simulink model "hydraulicCylinder_1"  (R2025b)
settings: Solver=VariableStepAuto  StartTime=0.0  StopTime=30  RelTol=1e-3
InitFcn:
  | hyd_parameter
undefined symbols (not defined in the file or in its folder): cyl, valve
libraries: SignalEditorBlockLib x3, slpidlib x1, simulink x1
settings Model: LastModifiedBy=binh.le

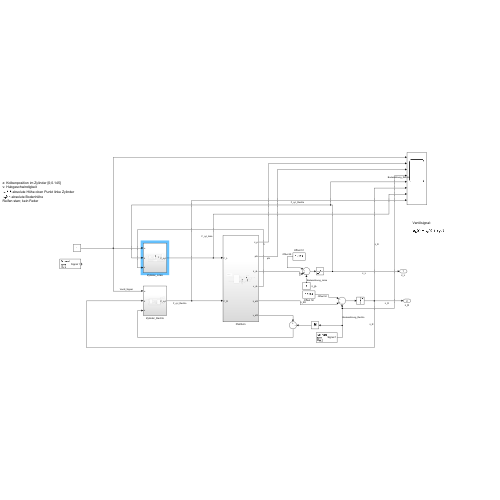
[thumbnail: Simulink's stored preview of the top-level diagram]
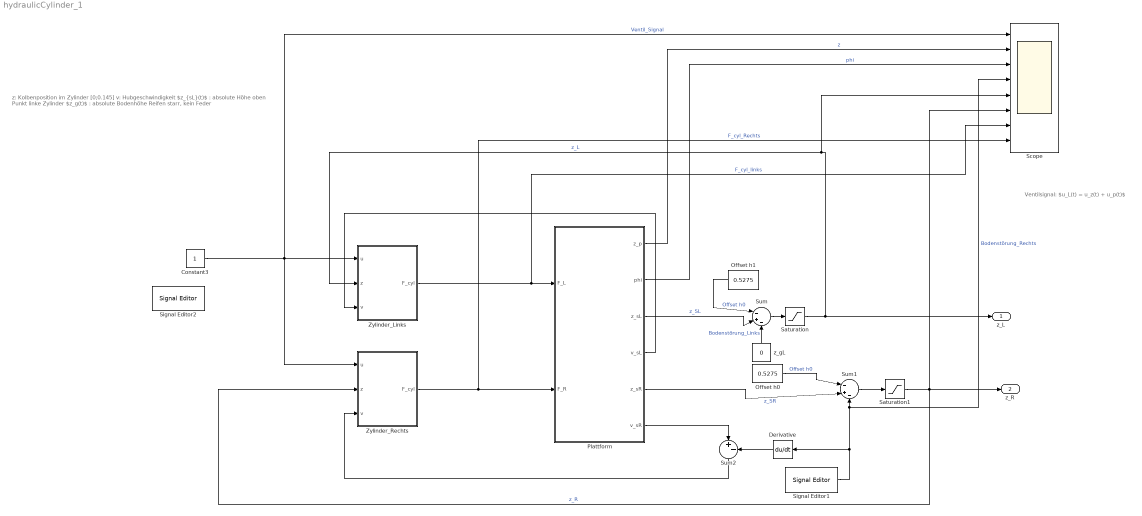
== system hydraulicCylinder_1 ==
  note: z: Kolbenposition im Zylinder [0;0.145]
      | v: Hubgeschwindigkeit
      | $z_{sL}(t)$ : absolute Höhe oben Punkt linke Zylinder
      | $z_g(t)$ : absolute Bodenhöhe
      | Reifen starr, kein Feder
  note: Ventilsignal:
      |
      | $u_L(t) = u_z(t) + u_p(t)$
  Constant3 : Constant
  Derivative : Derivative
  Offset h0 : Constant  Value=0.5275
  Offset h1 : Constant  Value=0.5275
  Plattform : Subsystem
  Saturation : Saturate  UpperLimit=0.145  LowerLimit=0
  Saturation1 : Saturate  UpperLimit=0.145  LowerLimit=0
  Scope : Scope  NumInputPorts=8
      settings: ActiveDisplayString=7  ActiveDisplayYMinimum=-28869.174120408497  ActiveDisplayYMaximum=66545.684568252938
  Signal Editor1 : SignalEditorBlockLib/Signal Editor  FileName=W:\BINH_MATLAB\bodenstörung.mat  ActiveScenario=Scenario  ActiveSignal=Signal 1  IsBus=off  OutputBusObjectStr=Bus: BusObject  SampleTime=0  ZeroCross=off  OutputAfterFinalValue=Setting to zero  Unit=inherit  PreserveSignalName=on  ApplySigPropsToAllScenarios=on  ApplySigPropsToAllSignals=off  SignalPropertySource=Dialog parameters
  Signal Editor2 : SignalEditorBlockLib/Signal Editor  FileName=signal.mat  ActiveScenario=Scenario  ActiveSignal=Signal 1  IsBus=off  OutputBusObjectStr=Bus: BusObject  SampleTime=0  ZeroCross=off  OutputAfterFinalValue=Setting to zero  Unit=inherit  PreserveSignalName=on  ApplySigPropsToAllScenarios=on  ApplySigPropsToAllSignals=off  SignalPropertySource=Dialog parameters
  Sum : Sum  Inputs=|-+-
  Sum1 : Sum  Inputs=|-+-
  Sum2 : Sum  Inputs=|+-
  Zylinder_Links : Subsystem
  Zylinder_Rechts : Subsystem
  z_gL : Constant  Value=0
  z_L : Outport
  z_R : Outport  Port=2
  wires:
  Zylinder_Links/1(F_cyl) -> Scope/7, Plattform/1(F_L)  "F_cyl_links"
  Zylinder_Rechts/1(F_cyl) -> Scope/8, Plattform/2(F_R)  "F_cyl_Rechts"
  Plattform/3(z_sL) -> Sum/2  "z_SL"
  z_gL/1 -> Sum/3  "Bodenstörung_Links"
  Sum/1 -> Saturation/1
  Constant3/1 -> Zylinder_Rechts/1(u), Scope/1, Zylinder_Links/1(u)  "Ventil_Signal"
  Plattform/1(z_p) -> Scope/2  "z"
  Plattform/2(phi) -> Scope/3  "phi"
  Plattform/5(z_sR) -> Sum1/2  "z_SR"
  Sum1/1 -> Saturation1/1
  Plattform/4(v_sL) -> Zylinder_Links/3(v)
  Saturation/1 -> Scope/5, Zylinder_Links/2(z), z_L/1  "z_L"
  Saturation1/1 -> Scope/6, Zylinder_Rechts/2(z), z_R/1  "z_R"
  Signal Editor1/1 -> Derivative/1, Scope/4, Sum1/3  "Bodenstörung_Rechts"
  Derivative/1 -> Sum2/2
  Plattform/6(v_sR) -> Sum2/1
  Sum2/1 -> Zylinder_Rechts/3(v)
  Offset h0/1 -> Sum1/1  "Offset h0"
  Offset h1/1 -> Sum/1  "Offset h0"

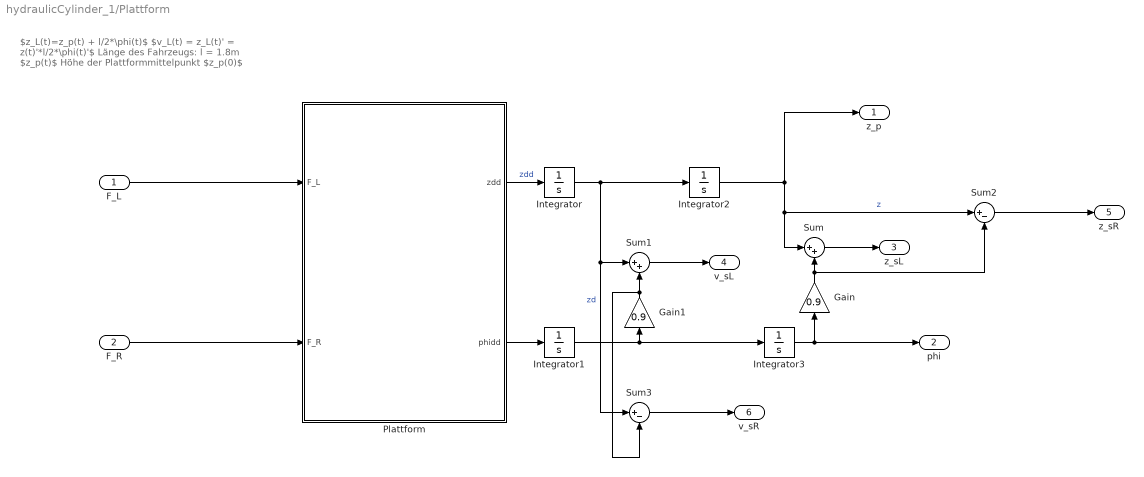
== system hydraulicCylinder_1/Plattform ==
  note: $z_L(t)=z_p(t) + l/2*\phi(t)$
      | $v_L(t) = z_L(t)' = z(t)'*l/2*\phi(t)'$
      | Länge des Fahrzeugs: l = 1.8m
      | $z_p(t)$ Höhe der Plattformmittelpunkt
      | $z_p(0)$
  F_L : Inport
  F_R : Inport  Port=2
  Gain : Gain  Gain=0.9
  Gain1 : Gain  Gain=0.9
  Integrator : Integrator
  Integrator1 : Integrator
  Integrator2 : Integrator  InitialCondition=0.6
  Integrator3 : Integrator
  Plattform : MATLAB Function  TreatAsAtomicUnit=on
  Sum : Sum  Inputs=|++
  Sum1 : Sum  Inputs=|++
  Sum2 : Sum  Inputs=|+-
  Sum3 : Sum  Inputs=|+-
  z_p : Outport
  phi : Outport  Port=2
  z_sL : Outport  Port=3
  v_sL : Outport  Port=4
  z_sR : Outport  Port=5
  v_sR : Outport  Port=6
  wires:
  Integrator/1 -> Sum3/1, Sum1/1, Integrator2/1  "zd"
  Integrator2/1 -> Sum/1, Sum2/1, z_p/1  "z"
  Plattform/2(phidd) -> Integrator1/1
  Plattform/1(zdd) -> Integrator/1  "zdd"
  F_L/1 -> Plattform/1(F_L)
  Integrator1/1 -> Gain1/1, Integrator3/1
  F_R/1 -> Plattform/2(F_R)
  Integrator3/1 -> phi/1, Gain/1
  Gain/1 -> Sum2/2, Sum/2
  Sum/1 -> z_sL/1
  Gain1/1 -> Sum3/2, Sum1/2
  Sum1/1 -> v_sL/1
  Sum2/1 -> z_sR/1
  Sum3/1 -> v_sR/1

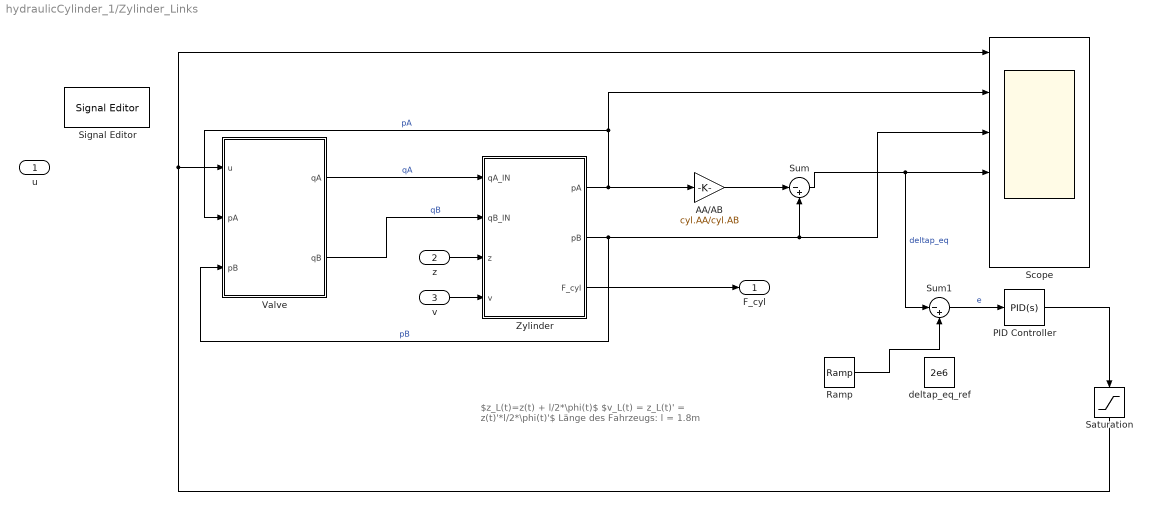
== system hydraulicCylinder_1/Zylinder_Links ==
  note: $z_L(t)=z(t) + l/2*\phi(t)$
      | $v_L(t) = z_L(t)' = z(t)'*l/2*\phi(t)'$
      | Länge des Fahrzeugs: l = 1.8m
  u : Inport
  z : Inport  Port=2
  v : Inport  Port=3
  AA/AB : Gain  Gain=cyl.AA/cyl.AB
  PID Controller : slpidlib/PID Controller  Controller=PID  Form=Parallel  TimeDomain=Continuous-time  UseExternalTs=off  SampleTime=-1  IntegratorMethod=Forward Euler  FilterMethod=Forward Euler  ControllerParametersSource=internal  P=4e-7  I=1e-7  UseKiTs=off  D=0  UseExternalDerivativeSource=off  N=100  UseFilter=on  TunerSelectOption=Transfer Function Based (PID Tuner App)  InitialConditionSource=internal  InitialConditionForIntegrator=0  InitialConditionForFilter=0  DifferentiatorICPrevScaledInput=0  ExternalReset=none  TrackingMode=off  Kt=1  LimitOutput=on  SatLimitsSource=internal  UpperSaturationLimit=1  LowerSaturationLimit=-1  LinearizeAsGain=on  AntiWindupMode=back-calculation  Kb=50  LimitIntegrator=off  UpperIntegratorSaturationLimit=inf  LowerIntegratorSaturationLimit=-inf  POutMin=[]  POutMax=[]  IOutMin=[]  IOutMax=[]  DOutMin=[]  DOutMax=[]  NOutMin=[]  NOutMax=[]  SumOutMin=[]  SumOutMax=[]  SaturationOutMin=[]  SaturationOutMax=[]  PParamMin=[]  PParamMax=[]  IParamMin=[]  IParamMax=[]  DParamMin=[]  DParamMax=[]  NParamMin=[]  NParamMax=[]  KbParamMin=[]  KbParamMax=[]  KtParamMin=[]  KtParamMax=[]  KbOutMin=[]  KbOutMax=[]  KtOutMin=[]  KtOutMax=[]  IntegratorOutMin=[]  IntegratorOutMax=[]  FilterOutMin=[]  FilterOutMax=[]  SumI1OutMin=[]  SumI1OutMax=[]  SumI2OutMin=[]  SumI2OutMax=[]  SumI3OutMin=[]  SumI3OutMax=[]  SumI4OutMin=[]  SumI4OutMax=[]  SumDOutMin=[]  SumDOutMax=[]  DifferentiatorOutMin=[]  DifferentiatorOutMax=[]  FilterDiffOutCoefMin=[]  FilterDiffOutCoefMax=[]  ReciprocalOutMin=[]  ReciprocalOutMax=[]  SumDenOutMin=[]  SumDenOutMax=[]  SumNumOutMin=[]  SumNumOutMax=[]  DivideOutMin=[]  DivideOutMax=[]  UdiffTsProdOutMin=[]  UdiffTsProdOutMax=[]  NTsProdOutMin=[]  NTsProdOutMax=[]  UintegralTsProdOutMin=[]  UintegralTsProdOutMax=[]  UngainTsProdOutMin=[]  UngainTsProdOutMax=[]  ClampingZeroOutDataTypeStr=Inherit: Inherit via back propagation  ClampingZeroOutMin=[]  ClampingZeroOutMax=[]  FilterDenConstantOutDataTypeStr=Inherit: Inherit via back propagation  FilterDenConstantOutMin=[]  FilterDenConstantOutMax=[]  PCopyOutDataTypeStr=Inherit: Inherit via back propagation  PCopyOutMin=[]  PCopyOutMax=[]  NCopyOutDataTypeStr=Inherit: Inherit via back propagation  NCopyOutMin=[]  NCopyOutMax=[]  IntegratorContinuousStateAttributes=''  IntegratorStateMustResolveToSignalObject=off  IntegratorRTWStateStorageClass=Auto  FilterContinuousStateAttributes=''  FilterStateMustResolveToSignalObject=off  FilterRTWStateStorageClass=Auto  ParallelPVariant=InternalParameters  IdealPVariant=Disabled  IVariant=InternalParameters  DVariant=InternalParameters  IntegratorVariant=Continuous  SatVariant=Enabled  AWVariant=BackCalculation  PCopyVariant=Disabled  TRVariant=Disabled  FdbkBlocksVariant=Forward  IdealPFdbkVariant=Disabled  SatFdbkVariant=Disabled  DerivativeFilterVariant=ContFilter  NVariant=InternalParameters  NCopyVariant=Disabled  FilterICVariant=InternalICsFilter  IntegratorICVariant=InternalICs  ExternalResetVariant=Disabled  TRSumVariant=Passthrough  SumFdbkVariant=Disabled  SumVariant=Sum_PID  TsampFilterVariant=InternalTs  TsampNgainVariant=Passthrough  TsampIntegralVariant=Disabled_SignalSpec  ExternalSaturationOutDataTypeStr=Inherit: Same as second input  DerivativeSourceVariant=ErrorSignal  PreIntVariant=InternalPreInt
  Ramp : simulink/Sources/Ramp  slope=2e6  start=2  InitialOutput=0
  Saturation : Saturate  UpperLimit=1  LowerLimit=-1
  Scope : Scope  NumInputPorts=6
      settings: ActiveDisplayYMinimum=-1.25  ActiveDisplayYMaximum=1.25
  Signal Editor : SignalEditorBlockLib/Signal Editor  FileName=signal.mat  ActiveScenario=Scenario  ActiveSignal=Signal 1  IsBus=off  OutputBusObjectStr=Bus: BusObject  SampleTime=0  ZeroCross=off  OutputAfterFinalValue=Setting to zero  Unit=inherit  PreserveSignalName=on  ApplySigPropsToAllScenarios=on  ApplySigPropsToAllSignals=off  SignalPropertySource=Dialog parameters
  Sum : Sum  Inputs=|-+
  Sum1 : Sum  Inputs=|-+
  Valve : Subsystem
  Zylinder : Subsystem
  deltap_eq_ref : Constant  Value=2e6
  F_cyl : Outport
  wires:
  PID Controller/1 -> Saturation/1
  z/1 -> Zylinder/3(z)
  Zylinder/2(pB) -> Sum/2, Scope/3, Valve/3(pB)  "pB"
  v/1 -> Zylinder/4(v)
  Zylinder/3(F_cyl) -> F_cyl/1
  Zylinder/1(pA) -> Valve/2(pA), Scope/2, AA/AB/1  "pA"
  Valve/1(qA) -> Zylinder/1(qA_IN)  "qA"
  Valve/2(qB) -> Zylinder/2(qB_IN)  "qB"
  Sum/1 -> Scope/4, Sum1/1  "deltap_eq"
  AA/AB/1 -> Sum/1
  Ramp/1 -> Sum1/2
  Sum1/1 -> PID Controller/1  "e"
  Saturation/1 -> Scope/1, Valve/1(u)

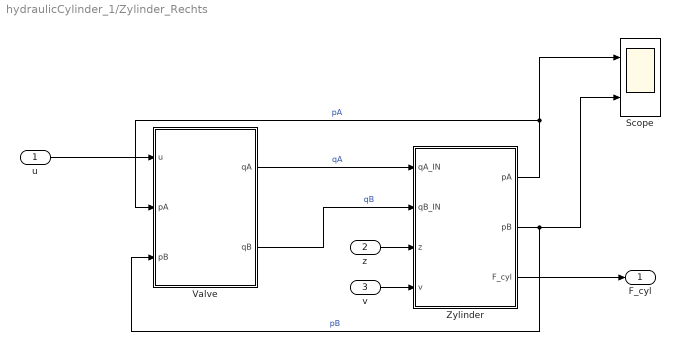
== system hydraulicCylinder_1/Zylinder_Rechts ==
  u : Inport
  z : Inport  Port=2
  v : Inport  Port=3
  Scope : Scope  NumInputPorts=2
      settings: ActiveDisplayYMinimum=-1  ActiveDisplayYMaximum=1  DataLoggingVariableName=ScopeData2
  Valve : Subsystem
  Zylinder : Subsystem
  F_cyl : Outport
  wires:
  u/1 -> Valve/1(u)
  z/1 -> Zylinder/3(z)
  Zylinder/2(pB) -> Scope/2, Valve/3(pB)  "pB"
  v/1 -> Zylinder/4(v)
  Zylinder/3(F_cyl) -> F_cyl/1
  Zylinder/1(pA) -> Scope/1, Valve/2(pA)  "pA"
  Valve/1(qA) -> Zylinder/1(qA_IN)  "qA"
  Valve/2(qB) -> Zylinder/2(qB_IN)  "qB"

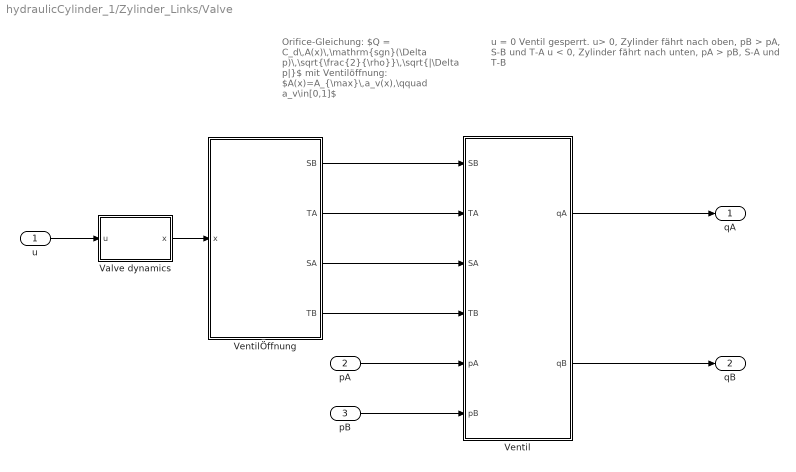
== system hydraulicCylinder_1/Zylinder_Links/Valve ==
  note: Orifice-Gleichung:
      | $Q = C_d\,A(x)\,\mathrm{sgn}(\Delta p)\,\sqrt{\frac{2}{\rho}}\,\sqrt{|\Delta p|}$
      | mit Ventilöffnung:
      | $A(x)=A_{\max}\,a_v(x),\qquad a_v\in[0,1]$
  note: u = 0 Ventil gesperrt.
      | u> 0, Zylinder fährt nach oben, pB > pA, S-B und T-A
      | u < 0, Zylinder fährt nach unten, pA > pB, S-A und T-B
  u : Inport
  pA : Inport  Port=2
  pB : Inport  Port=3
  Valve dynamics : Subsystem
  Ventil : MATLAB Function  TreatAsAtomicUnit=on
  VentilÖffnung : MATLAB Function  TreatAsAtomicUnit=on
  qA : Outport
  qB : Outport  Port=2
  wires:
  Ventil/1(qA) -> qA/1
  Ventil/2(qB) -> qB/1
  pB/1 -> Ventil/6(pB)
  pA/1 -> Ventil/5(pA)
  u/1 -> Valve dynamics/1(u)
  Valve dynamics/1(x) -> VentilÖffnung/1(x)
  VentilÖffnung/3(SA) -> Ventil/3(SA)
  VentilÖffnung/2(TA) -> Ventil/2(TA)
  VentilÖffnung/1(SB) -> Ventil/1(SB)
  VentilÖffnung/4(TB) -> Ventil/4(TB)

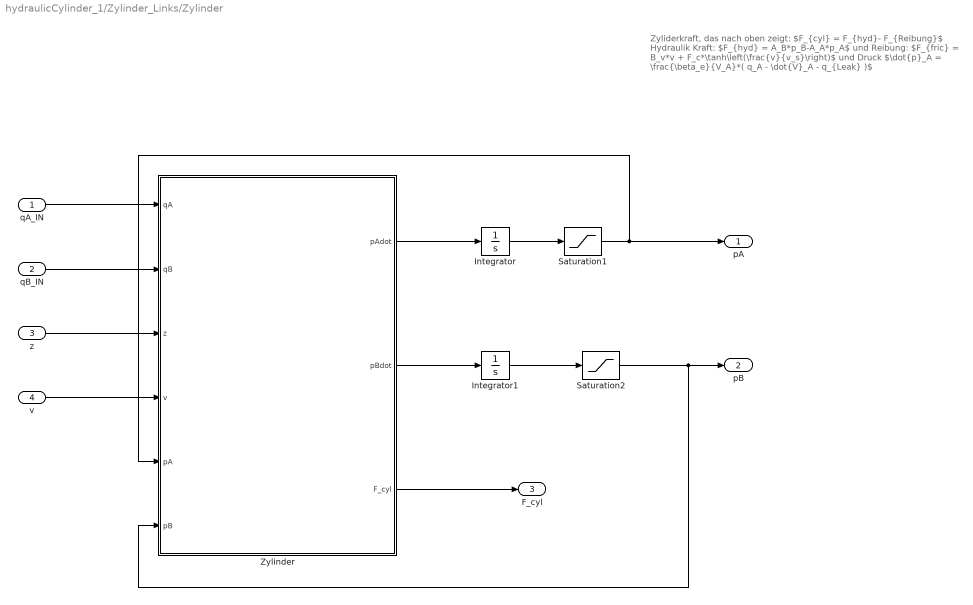
== system hydraulicCylinder_1/Zylinder_Links/Zylinder ==
  note: Zyliderkraft, das nach oben zeigt:
      | $F_{cyl} = F_{hyd}- F_{Reibung}$
      | Hydraulik Kraft:
      | $F_{hyd} = A_B*p_B-A_A*p_A$
      | und Reibung:
      | $F_{fric} = B_v*v + F_c*\tanh\left(\frac{v}{v_s}\right)$
      | und Druck
      | $\dot{p}_A = \frac{\beta_e}{V_A}*( q_A - \dot{V}_A - q_{Leak} )$
  qA_IN : Inport
  qB_IN : Inport  Port=2
  z : Inport  Port=3
  v : Inport  Port=4
  Integrator : Integrator  InitialCondition=valve.pT
  Integrator1 : Integrator  InitialCondition=9e6
  Saturation1 : Saturate  UpperLimit=cyl.pMax  LowerLimit=cyl.pMin
  Saturation2 : Saturate  UpperLimit=cyl.pMax  LowerLimit=cyl.pMin
  Zylinder : MATLAB Function  TreatAsAtomicUnit=on
  pA : Outport
  pB : Outport  Port=2
  F_cyl : Outport  Port=3
  wires:
  v/1 -> Zylinder/4(v)
  z/1 -> Zylinder/3(z)
  qA_IN/1 -> Zylinder/1(qA)
  qB_IN/1 -> Zylinder/2(qB)
  Zylinder/1(pAdot) -> Integrator/1
  Zylinder/2(pBdot) -> Integrator1/1
  Zylinder/3(F_cyl) -> F_cyl/1
  Integrator/1 -> Saturation1/1
  Integrator1/1 -> Saturation2/1
  Saturation1/1 -> Zylinder/5(pA), pA/1
  Saturation2/1 -> Zylinder/6(pB), pB/1

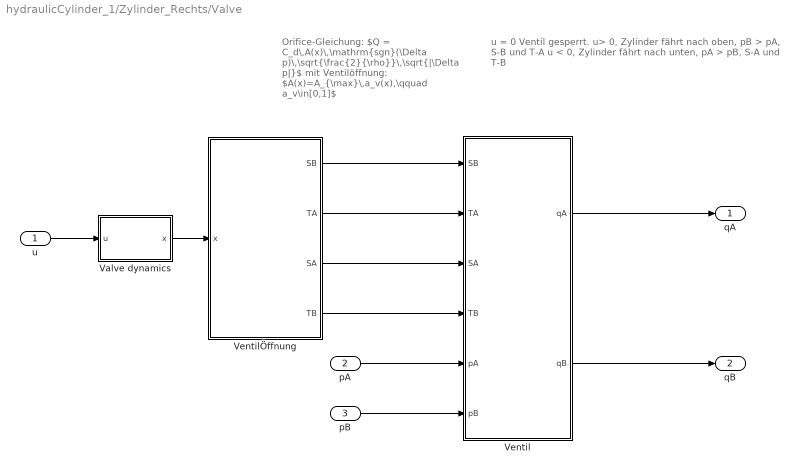
== system hydraulicCylinder_1/Zylinder_Rechts/Valve ==
  note: Orifice-Gleichung:
      | $Q = C_d\,A(x)\,\mathrm{sgn}(\Delta p)\,\sqrt{\frac{2}{\rho}}\,\sqrt{|\Delta p|}$
      | mit Ventilöffnung:
      | $A(x)=A_{\max}\,a_v(x),\qquad a_v\in[0,1]$
  note: u = 0 Ventil gesperrt.
      | u> 0, Zylinder fährt nach oben, pB > pA, S-B und T-A
      | u < 0, Zylinder fährt nach unten, pA > pB, S-A und T-B
  u : Inport
  pA : Inport  Port=2
  pB : Inport  Port=3
  Valve dynamics : Subsystem
  Ventil : MATLAB Function  TreatAsAtomicUnit=on
  VentilÖffnung : MATLAB Function  TreatAsAtomicUnit=on
  qA : Outport
  qB : Outport  Port=2
  wires:
  Ventil/1(qA) -> qA/1
  Ventil/2(qB) -> qB/1
  pB/1 -> Ventil/6(pB)
  pA/1 -> Ventil/5(pA)
  u/1 -> Valve dynamics/1(u)
  Valve dynamics/1(x) -> VentilÖffnung/1(x)
  VentilÖffnung/3(SA) -> Ventil/3(SA)
  VentilÖffnung/2(TA) -> Ventil/2(TA)
  VentilÖffnung/1(SB) -> Ventil/1(SB)
  VentilÖffnung/4(TB) -> Ventil/4(TB)

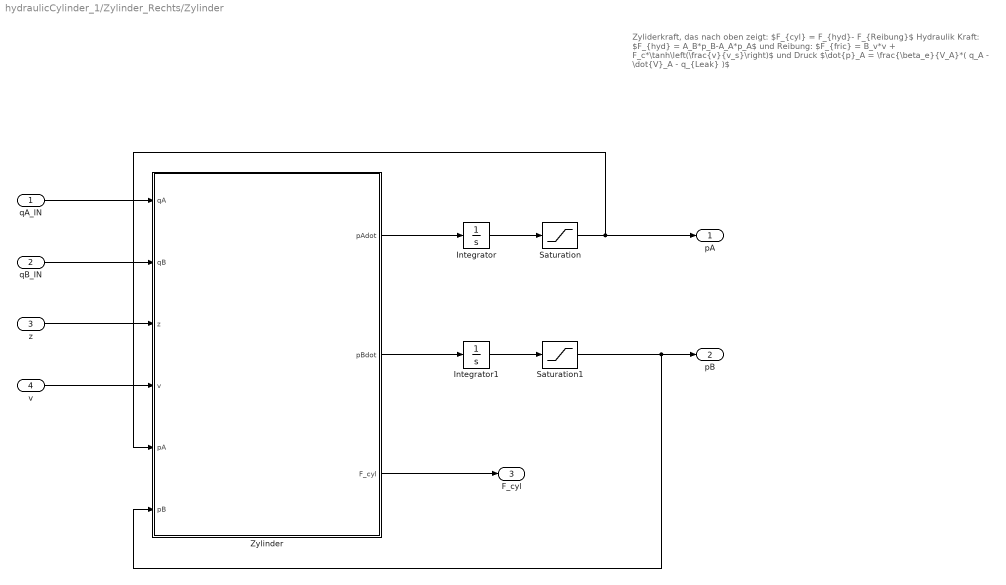
== system hydraulicCylinder_1/Zylinder_Rechts/Zylinder ==
  note: Zyliderkraft, das nach oben zeigt:
      | $F_{cyl} = F_{hyd}- F_{Reibung}$
      | Hydraulik Kraft:
      | $F_{hyd} = A_B*p_B-A_A*p_A$
      | und Reibung:
      | $F_{fric} = B_v*v + F_c*\tanh\left(\frac{v}{v_s}\right)$
      | und Druck
      | $\dot{p}_A = \frac{\beta_e}{V_A}*( q_A - \dot{V}_A - q_{Leak} )$
  qA_IN : Inport
  qB_IN : Inport  Port=2
  z : Inport  Port=3
  v : Inport  Port=4
  Integrator : Integrator  InitialCondition=valve.pT
  Integrator1 : Integrator  InitialCondition=9e6
  Saturation : Saturate  UpperLimit=cyl.pMax  LowerLimit=cyl.pMin
  Saturation1 : Saturate  UpperLimit=cyl.pMax  LowerLimit=cyl.pMin
  Zylinder : MATLAB Function  TreatAsAtomicUnit=on
  pA : Outport
  pB : Outport  Port=2
  F_cyl : Outport  Port=3
  wires:
  v/1 -> Zylinder/4(v)
  z/1 -> Zylinder/3(z)
  qA_IN/1 -> Zylinder/1(qA)
  qB_IN/1 -> Zylinder/2(qB)
  Zylinder/1(pAdot) -> Integrator/1
  Integrator/1 -> Saturation/1
  Zylinder/2(pBdot) -> Integrator1/1
  Integrator1/1 -> Saturation1/1
  Zylinder/3(F_cyl) -> F_cyl/1
  Saturation/1 -> Zylinder/5(pA), pA/1
  Saturation1/1 -> Zylinder/6(pB), pB/1

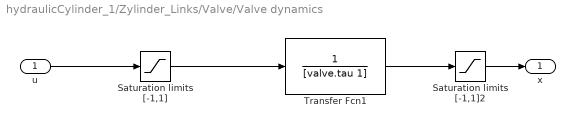
== system hydraulicCylinder_1/Zylinder_Links/Valve/Valve dynamics ==
  u : Inport
  Saturation limits [-1,1] : Saturate  UpperLimit=1  LowerLimit=-1
  Saturation limits [-1,1]2 : Saturate  UpperLimit=1  LowerLimit=-1
  Transfer Fcn1 : TransferFcn  Denominator=[valve.tau 1]
  x : Outport  VectorParamsAs1DForOutWhenUnconnected=off
  wires:
  u/1 -> Saturation limits [-1,1]/1
  Transfer Fcn1/1 -> Saturation limits [-1,1]2/1
  Saturation limits [-1,1]2/1 -> x/1
  Saturation limits [-1,1]/1 -> Transfer Fcn1/1

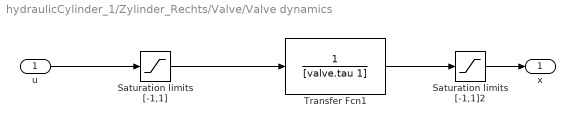
== system hydraulicCylinder_1/Zylinder_Rechts/Valve/Valve dynamics ==
  u : Inport
  Saturation limits [-1,1] : Saturate  UpperLimit=1  LowerLimit=-1
  Saturation limits [-1,1]2 : Saturate  UpperLimit=1  LowerLimit=-1
  Transfer Fcn1 : TransferFcn  Denominator=[valve.tau 1]
  x : Outport  VectorParamsAs1DForOutWhenUnconnected=off
  wires:
  u/1 -> Saturation limits [-1,1]/1
  Transfer Fcn1/1 -> Saturation limits [-1,1]2/1
  Saturation limits [-1,1]2/1 -> x/1
  Saturation limits [-1,1]/1 -> Transfer Fcn1/1

== matlab function hydraulicCylinder_1/Plattform/Plattform ==
  data: zdd output; phidd output; F_L input; F_R input
function [zdd, phidd] = platform_2dof(F_L, F_R)
g   = 9.81;
m_total = 6000;
m_s = m_total/3;    
l   = 1.8;           

Jphi = m_s * l^2 / 12;


zdd = (F_L + F_R - m_s * g) / m_s;


phidd = ( (l/2)*F_L - (l/2)*F_R ) / Jphi;


end

== matlab function hydraulicCylinder_1/Zylinder_Links/Zylinder/Zylinder ==
  data: pAdot output; pBdot output; qA input; F_cyl output; qB input; z input; v input; pA input; pB input
function [pAdot,pBdot,F_cyl] = cylinder(qA,qB,z,v,pA,pB)
cyl.D = 0.09; % m datenblatt
cyl.d = 0.07; %m datenblatt
cyl.AB  =pi*0.09^2/4;       % m^2 (Kolbenseite) datenblatt
cyl.AA  = pi*(0.09^2-0.07^2)/4;       % m^2 (Stangenseite)  datenblatt
cyl.L   = 0.145;          % m datenblatt
cyl.VA0 = 2e-4;         % m^3 geschätzt
cyl.VB0 = 2e-4;         % m^3 geschätzt
cyl.Vmin = 1e-5;        % m^3 geschätzt
cyl.be  = 1e9;          % Pa (Bulkmodul) geschätzt
cyl.CL  = 1e-12;        % m^3/(s*Pa) Leckage A<->B geschätzt

% friction
cyl.Bv = 1500;          % N*s/m geschätzt
cyl.Fc = 1500;           % N geschätzt
cyl.vs = 1e-3;          % m/s smoothing geschätzt
cyl.pMin = 1e5;         % Pa (Kavitation vermeiden) geschätzt
cyl.pMax = 2e7;         % Pa datenblatt

% volumes
VA = max(cyl.Vmin, cyl.VA0 + cyl.AA * (cyl.L- z));
VB = max(cyl.Vmin, cyl.VB0 + cyl.AB * z);

% leakage (A -> B positive)
qLeak = cyl.CL * (pA - pB);

% dp = (be/V)*(Qin - dVdt +/- leakage)
VAdot = -cyl.AA * v;
VBdot = cyl.AB * v;

pAdot = (cyl.be / VA) * ( qA - VAdot - qLeak );
pBdot = (cyl.be / VB) * ( qB - VBdot + qLeak );


% hydraulik Kraft
F_hyd = cyl.AB * pB - cyl.AA * pA;

% Reibung
F_fric = cyl.Bv * v + cyl.Fc * tanh(v / cyl.vs);

F_cyl = F_hyd - F_fric;
end

== matlab function hydraulicCylinder_1/Zylinder_Links/Valve/Ventil ==
  data: SB input; TA input; SA input; TB input; pA input; pB input; qA output; qB output
function [qA, qB] = valve_portflows(SB, TA, SA, TB, pA, pB)
% Eingänge:
%   SA, TA, SB, TB : relative Öffnungen [0..1]
%       SA = P(Supply) -> A
%       TA = A -> T(Tank)
%       SB = P(Supply) -> B
%       TB = B -> T(Tank)
%   pA, pB         : Kammerdrücke
%
% Ausgänge:
%   qA, qB         : Netto-Volumenstrom IN die Kammern A/B 
%                   (positiv bedeutet: Zufluss in die Kammer)

%Parameter
pS   = 14e6;    % Versorgungsdruck [Pa] (z.B. Datenblatt)
pT   = 1e5;     % Tankdruck [Pa]
rho  = 850;     % Dichte [kg/m^3]
Cd   = 0.62;    % Durchflusskoeffizient [-]
Amax = 3e-6;    % maximale Orifice-Fläche [m^2] (Schätzwert)
dp_eps = 50;    % Totband für Druckdifferenz [Pa] (gegen numerisches Rauschen)

% Öffnungen sicher auf [0..1] begrenzen
SA = min(max(SA, 0), 1);
TA = min(max(TA, 0), 1);
SB = min(max(SB, 0), 1);
TB = min(max(TB, 0), 1);

% Einzelströme der vier Kanten
qSA = orifice(pS, pA, SA, Cd, Amax, rho, dp_eps);  % P -> A
qTA = orifice(pA, pT, TA, Cd, Amax, rho, dp_eps);  % A -> T
qSB = orifice(pS, pB, SB, Cd, Amax, rho, dp_eps);  % P -> B
qTB = orifice(pB, pT, TB, Cd, Amax, rho, dp_eps);  % B -> T

% Nettozufluss in die Kammern: Zufluss aus Versorgung minus Abfluss zum Tank
qA = qSA - qTA;
qB = qSB - qTB;
end

function q = orifice(p_up, p_dn, a_rel, Cd, Amax, rho, dp_eps)
% Orifice-Gleichung (bidirektional):
% q = Cd * A * sign(dp) * sqrt(2/rho) * sqrt(|dp|)
% Damit ist auch Rückströmung möglich, falls p_dn > p_up.

A  = Amax * a_rel;
dp = p_up - p_dn;

% kleines Totband um dp=0, damit bei fast gleichen Drücken nicht "zittert"
if abs(dp) < dp_eps || A <= 0
    q = 0;
    return;
end

q = Cd * A * sign(dp) * sqrt(2/rho) * sqrt(abs(dp));
end

== matlab function hydraulicCylinder_1/Zylinder_Links/Valve/VentilÖffnung ==
  data: SB output; TA output; x input; SA output; TB output
function [SB, TA, SA, TB] = relative_opening(x)
% 4/3-Proportionalventil:
% Eingabe x in [-1..1] -> relative Öffnungen SA, SB, TA, TB in [0..1]
%   SA: P(Supply) -> A
%   SB: P(Supply) -> B
%   TA: A -> T(Tank)
%   TB: B -> T(Tank)
% Ventil-Parameter (typische Startwerte für Proportionalventil)
valve.udz = 0.05;   % Totzone (5%) um Nullstellung

% Stützstellen für |x| nach Totzone-Normierung -> Bereich [0..1]
valve.bp  = [0    0.05  0.10  0.20  0.35  0.50  0.70  1.00];

% Kennlinie: relative Öffnung (sanfter Start, danach ungefähr linear)
valve.tbl = [0    0.01  0.04  0.12  0.28  0.50  0.78  1.00];

% Für den Anfang symmetrisch: alle vier Kanten bekommen die gleiche Kennlinie
valve.tbl_SA = [0    0.01  0.04  0.12  0.28  0.50  0.78  1.00];
valve.tbl_SB = [0    0.01  0.04  0.12  0.28  0.50  0.78  1.00];
valve.tbl_TA = [0    0.01  0.04  0.12  0.28  0.50  0.78  1.00];
valve.tbl_TB = [0    0.01  0.04  0.12  0.28  0.50  0.78  1.00];

%Sicherheit: Eingang auf zulässigen Bereich begrenzen
x = min(max(x, -1), 1);

%Aufteilen in positiven/negativen Anteil
xp = max(x, 0);      % Betrag für x > 0
xn = max(-x, 0);     % Betrag für x < 0  (als positiver Wert)

%Totzone anwenden und danach auf [0..1] normieren
% Damit gilt: x = 1  -> 1,  und |x| <= udz -> 0
xp = deadzone_norm(xp, valve.udz);
xn = deadzone_norm(xn, valve.udz);

%   x > 0 -> SB und TA öffnen
%   x < 0 -> SA und TB öffnen
SB = lookup1d(xp, valve.bp, valve.tbl_SB);
TA = lookup1d(xp, valve.bp, valve.tbl_TA);

SA = lookup1d(xn, valve.bp, valve.tbl_SA);
TB = lookup1d(xn, valve.bp, valve.tbl_TB);

%Öffnungen auf [0..1] begrenzen
SA = min(max(SA, 0), 1);
SB = min(max(SB, 0), 1);
TA = min(max(TA, 0), 1);
TB = min(max(TB, 0), 1);
end

function y = deadzone_norm(x, dz)
% Totzone + Normierung
% x ist bereits >= 0
% Wenn x <= dz -> 0
% Sonst skaliert auf (0..1): (x-dz)/(1-dz)
if x <= dz
    y = 0;
else
    y = (x - dz) / (1 - dz);
end
end

function y = lookup1d(x, bp, tbl)
% Einfache 1D Lookup-Tabelle (stückweise linear) mit Begrenzung von x
n = numel(bp);

% Sicherheitscheck: bp und tbl müssen gleich lang sein
if numel(tbl) ~= n
    y = 0;
    return;
end

% x begrenzen (kein Extrapolieren)
x = min(max(x, bp(1)), bp(end));

% Default-Wert (falls numerische Randfälle)
y = tbl(end);
for i = 1:n-1
    if x >= bp(i) && x <= bp(i+1)
        den = (bp(i+1) - bp(i));
        if den <= 0
            y = tbl(i);
            return;
        end
        t = (x - bp(i)) / den;
        y = tbl(i) + t * (tbl(i+1) - tbl(i));
        return;
    end
end
end

== matlab function hydraulicCylinder_1/Zylinder_Rechts/Valve/Ventil ==
  data: SB input; TA input; SA input; TB input; pA input; pB input; qA output; qB output
function [qA, qB] = valve_portflows(SB, TA, SA, TB, pA, pB)
% Eingänge:
%   SA, TA, SB, TB : relative Öffnungen [0..1]
%       SA = P(Supply) -> A
%       TA = A -> T(Tank)
%       SB = P(Supply) -> B
%       TB = B -> T(Tank)
%   pA, pB         : Kammerdrücke
%
% Ausgänge:
%   qA, qB         : Netto-Volumenstrom IN die Kammern A/B 
%                   (positiv bedeutet: Zufluss in die Kammer)

%Parameter
pS   = 14e6;    % Versorgungsdruck [Pa] (z.B. Datenblatt)
pT   = 1e5;     % Tankdruck [Pa]
rho  = 850;     % Dichte [kg/m^3]
Cd   = 0.62;    % Durchflusskoeffizient [-]
Amax = 3e-6;    % maximale Orifice-Fläche [m^2] (Schätzwert)
dp_eps = 50;    % Totband für Druckdifferenz [Pa] (gegen numerisches Rauschen)

% Öffnungen sicher auf [0..1] begrenzen
SA = min(max(SA, 0), 1);
TA = min(max(TA, 0), 1);
SB = min(max(SB, 0), 1);
TB = min(max(TB, 0), 1);

% Einzelströme der vier Kanten
qSA = orifice(pS, pA, SA, Cd, Amax, rho, dp_eps);  % P -> A
qTA = orifice(pA, pT, TA, Cd, Amax, rho, dp_eps);  % A -> T
qSB = orifice(pS, pB, SB, Cd, Amax, rho, dp_eps);  % P -> B
qTB = orifice(pB, pT, TB, Cd, Amax, rho, dp_eps);  % B -> T

% Nettozufluss in die Kammern: Zufluss aus Versorgung minus Abfluss zum Tank
qA = qSA - qTA;
qB = qSB - qTB;
end

function q = orifice(p_up, p_dn, a_rel, Cd, Amax, rho, dp_eps)
% Orifice-Gleichung (bidirektional):
% q = Cd * A * sign(dp) * sqrt(2/rho) * sqrt(|dp|)
% Damit ist auch Rückströmung möglich, falls p_dn > p_up.

A  = Amax * a_rel;
dp = p_up - p_dn;

% kleines Totband um dp=0, damit bei fast gleichen Drücken nicht "zittert"
if abs(dp) < dp_eps || A <= 0
    q = 0;
    return;
end

q = Cd * A * sign(dp) * sqrt(2/rho) * sqrt(abs(dp));
end

== matlab function hydraulicCylinder_1/Zylinder_Rechts/Valve/VentilÖffnung ==
  data: SB output; TA output; x input; SA output; TB output
function [SB, TA, SA, TB] = relative_opening(x)
% 4/3-Proportionalventil:
% Eingabe x in [-1..1] -> relative Öffnungen SA, SB, TA, TB in [0..1]
%   SA: P(Supply) -> A
%   SB: P(Supply) -> B
%   TA: A -> T(Tank)
%   TB: B -> T(Tank)
% Ventil-Parameter (typische Startwerte für Proportionalventil)
valve.udz = 0.05;   % Totzone (5%) um Nullstellung

% Stützstellen für |x| nach Totzone-Normierung -> Bereich [0..1]
valve.bp  = [0    0.05  0.10  0.20  0.35  0.50  0.70  1.00];

% Kennlinie: relative Öffnung (sanfter Start, danach ungefähr linear)
valve.tbl = [0    0.01  0.04  0.12  0.28  0.50  0.78  1.00];

% Für den Anfang symmetrisch: alle vier Kanten bekommen die gleiche Kennlinie
valve.tbl_SA = [0    0.01  0.04  0.12  0.28  0.50  0.78  1.00];
valve.tbl_SB = [0    0.01  0.04  0.12  0.28  0.50  0.78  1.00];
valve.tbl_TA = [0    0.01  0.04  0.12  0.28  0.50  0.78  1.00];
valve.tbl_TB = [0    0.01  0.04  0.12  0.28  0.50  0.78  1.00];

%Sicherheit: Eingang auf zulässigen Bereich begrenzen
x = min(max(x, -1), 1);

%Aufteilen in positiven/negativen Anteil
xp = max(x, 0);      % Betrag für x > 0
xn = max(-x, 0);     % Betrag für x < 0  (als positiver Wert)

%Totzone anwenden und danach auf [0..1] normieren
% Damit gilt: x = 1  -> 1,  und |x| <= udz -> 0
xp = deadzone_norm(xp, valve.udz);
xn = deadzone_norm(xn, valve.udz);

%   x > 0 -> SB und TA öffnen
%   x < 0 -> SA und TB öffnen
SB = lookup1d(xp, valve.bp, valve.tbl_SB);
TA = lookup1d(xp, valve.bp, valve.tbl_TA);

SA = lookup1d(xn, valve.bp, valve.tbl_SA);
TB = lookup1d(xn, valve.bp, valve.tbl_TB);

%Öffnungen auf [0..1] begrenzen
SA = min(max(SA, 0), 1);
SB = min(max(SB, 0), 1);
TA = min(max(TA, 0), 1);
TB = min(max(TB, 0), 1);
end

function y = deadzone_norm(x, dz)
% Totzone + Normierung
% x ist bereits >= 0
% Wenn x <= dz -> 0
% Sonst skaliert auf (0..1): (x-dz)/(1-dz)
if x <= dz
    y = 0;
else
    y = (x - dz) / (1 - dz);
end
end

function y = lookup1d(x, bp, tbl)
% Einfache 1D Lookup-Tabelle (stückweise linear) mit Begrenzung von x
n = numel(bp);

% Sicherheitscheck: bp und tbl müssen gleich lang sein
if numel(tbl) ~= n
    y = 0;
    return;
end

% x begrenzen (kein Extrapolieren)
x = min(max(x, bp(1)), bp(end));

% Default-Wert (falls numerische Randfälle)
y = tbl(end);
for i = 1:n-1
    if x >= bp(i) && x <= bp(i+1)
        den = (bp(i+1) - bp(i));
        if den <= 0
            y = tbl(i);
            return;
        end
        t = (x - bp(i)) / den;
        y = tbl(i) + t * (tbl(i+1) - tbl(i));
        return;
    end
end
end

== matlab function hydraulicCylinder_1/Zylinder_Rechts/Zylinder/Zylinder ==
  data: pAdot output; pBdot output; qA input; F_cyl output; qB input; z input; v input; pA input; pB input
function [pAdot,pBdot,F_cyl] = cylinder(qA,qB,z,v,pA,pB)
% === Cylinder ===
cyl.D = 0.09; % m datenblatt
cyl.d = 0.07; %m datenblatt
cyl.AB  =pi*0.09^2/4;       % m^2 (Kolbenseite) datenblatt
cyl.AA  = pi*(0.09^2-0.07^2)/4;       % m^2 (Stangenseite)  datenblatt
cyl.L   = 0.145;          % m datenblatt
cyl.VA0 = 2e-4;         % m^3 geschätzt
cyl.VB0 = 2e-4;         % m^3 geschätzt
cyl.Vmin = 1e-5;        % m^3 geschätzt
cyl.be  = 1e9;          % Pa (Bulkmodul) geschätzt
cyl.CL  = 1e-12;        % m^3/(s*Pa) Leckage A<->B geschätzt

% friction
cyl.Bv = 1500;          % N*s/m geschätzt
cyl.Fc = 1500;           % N geschätzt
cyl.vs = 1e-3;          % m/s smoothing geschätzt
cyl.pMin = 1e5;         % Pa (Kavitation vermeiden) geschätzt
cyl.pMax = 2e7;         % Pa datenblatt

VA = max(cyl.Vmin, cyl.VA0 + cyl.AA * (cyl.L- z));
VB = max(cyl.Vmin, cyl.VB0 + cyl.AB * z);

% leakage (A -> B positive)
qLeak = cyl.CL * (pA - pB);

% dp = (be/V)*(Qin - dVdt +/- leakage)
VAdot = -cyl.AA * v;
VBdot = cyl.AB * v;

pAdot = (cyl.be / VA) * ( qA - VAdot - qLeak );
pBdot = (cyl.be / VB) * ( qB - VBdot + qLeak );


% hydraulik Kraft
F_hyd = cyl.AB * pB - cyl.AA * pA;

% Reibung
F_fric = cyl.Bv * v + cyl.Fc * tanh(v / cyl.vs);

F_cyl = F_hyd - F_fric;
end
